simulink model "AFC_FFNN_trainlm_15_15_15_15_Apr_1_2020"  (R2022b)
settings: Solver=ode15s  StartTime=0.0  StopTime=T  MaxStep=.01  RelTol=1e-3
undefined symbols (not defined in the file): AF_sensor_tol, fault_time, fuel_inj_tol, kappa_tol, MAF_sensor_tol, pump_tol, tau_ww_tol
libraries: neural x66
(part 2 of 3)

== system AFC_FFNN_trainlm_15_15_15_15_Apr_1_2020/Air Fuel Control Model 1/Feed-Forward Neural Network/Layer 2/Delays 1 ==
  "p{2}" : Inport  PortDimensions=15
      mask Display: e = 0.06;c1 = [120 230 180]/255;c2 = ([120 230 180]+0)/(256+128);c3 = ([120 230 180]+128)/(256+128);patch([0 1 1 0],[0 0 1 1],c1);patch([0 1 1 1-e 1-e 0+e],[0 0 1 1-e 0+e 0+e],c2);patch([0 0 1 1-e 0+e 0+e],[0 1 1 1-e 1-e 0+e],c3);plot([0 1 1 0 0],[0 0 1 1 0]);
  mux : Mux  Inputs=1
      mask Display: e = 0.06;c1 = [120 150 230]/255;c2 = ([120 150 230]+0)/383;c3 = ([120 150 230]+128)/383;patch([0 1 1 0],[0 0 1 1],c1);patch([0 1 1 1-e 1-e 0+e],[0 0 1 1-e 0+e 0+e],c2);patch([0 0 1 1-e 0+e 0+e],[0 1 1 1-e 1-e 0+e],c3);plot([0 1 1 0 0],[0 0 1 1 0]);disp('Mux')
  "pd{2,1}" : Outport
      mask Display: e = 0.06;c1 = [120 230 180]/255;c2 = ([120 230 180]+0)/(256+128);c3 = ([120 230 180]+128)/(256+128);patch([0 1 1 0],[0 0 1 1],c1);patch([0 1 1 1-e 1-e 0+e],[0 0 1 1-e 0+e 0+e],c2);patch([0 0 1 1-e 0+e 0+e],[0 1 1 1-e 1-e 0+e],c3);plot([0 1 1 0 0],[0 0 1 1 0]);
  wires:
  "p{2}"/1 -> mux/1
  mux/1 -> "pd{2,1}"/1

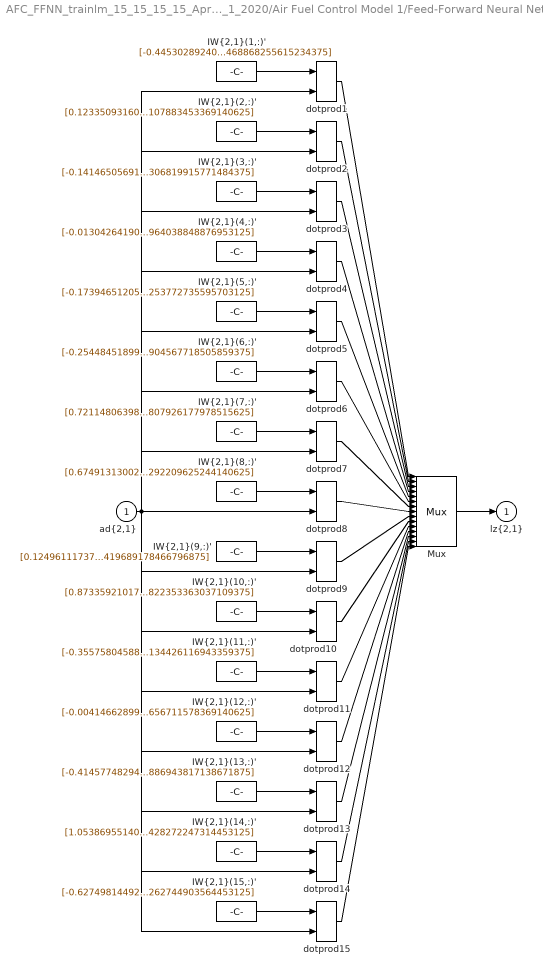
== system AFC_FFNN_trainlm_15_15_15_15_Apr_1_2020/Air Fuel Control Model 1/Feed-Forward Neural Network/Layer 2/LW{2,1} ==
  "ad{2,1}" : Inport  PortDimensions=15
      mask Display: e = 0.06;c1 = [120 230 180]/255;c2 = ([120 230 180]+0)/(256+128);c3 = ([120 230 180]+128)/(256+128);patch([0 1 1 0],[0 0 1 1],c1);patch([0 1 1 1-e 1-e 0+e],[0 0 1 1-e 0+e 0+e],c2);patch([0 0 1 1-e 0+e 0+e],[0 1 1 1-e 1-e 0+e],c3);plot([0 1 1 0 0],[0 0 1 1 0]);
  "IW{2,1}(1,:)'" : Constant  Value=[-0.44530289240325071631332320976071059703826904296875;-0.031599090975333421482673657010309398174285888671875;-0.9859158830932484018916284185252152383327484130859375;0.83077856260949634048529333085753023624420166015625;0.5147405056908984644081783699220977723598480224609375;-0.59941875528171539855293303844518959522247314453125;-0.9340218456622333409455904984497465193271636962890625;-0.2001276258897833615346684155156253837049007415771484375;0.08055251588838825693716927389687043614685535430908203125;-0.6770620370683728683758317856700159609317779541015625;0.318318052739778700743755734947626478970050811767578125;-0.51093086630106798740058593466528691351413726806640625;-0.44231337771352940979596723991562612354755401611328125;0.445164828909296483860913440366857685148715972900390625;0.9246634629628525114952708463533781468868255615234375]
      mask Display: e = 0.06;c1 = [120 150 230]/255;c2 = ([120 150 230]+0)/383;c3 = ([120 150 230]+128)/383;patch([0 1 1 0],[0 0 1 1],c1);patch([0 1 1 1-e 1-e 0+e],[0 0 1 1-e 0+e 0+e],c2);patch([0 0 1 1-e 0+e 0+e],[0 1 1 1-e 1-e 0+e],c3);plot([0 1 1 0 0],[0 0 1 1 0]);disp('weights');
  "IW{2,1}(10,:)'" : Constant  Value=[0.87335921017074824579395908585865981876850128173828125;0.3045430612282420401726312775281257927417755126953125;0.2262366289036867872397351675317622721195220947265625;-0.0737735854276786173766566889753448776900768280029296875;-0.63864720704534294615228873226442374289035797119140625;0.2937771056857114704286004780442453920841217041015625;0.56879031291023995908773258634028024971485137939453125;0.8502258695783304620618991975788958370685577392578125;0.59046290655221811416453192578046582639217376708984375;0.742343450952053895974813713110052049160003662109375;0.330116034595487717329120869180769659578800201416015625;0.422958081116346085170931701213703490793704986572265625;-0.5932782732724366514531766370055265724658966064453125;0.24289284049794712672110108542256057262420654296875;0.0864280836636444060872008776641450822353363037109375]
      mask Display: e = 0.06;c1 = [120 150 230]/255;c2 = ([120 150 230]+0)/383;c3 = ([120 150 230]+128)/383;patch([0 1 1 0],[0 0 1 1],c1);patch([0 1 1 1-e 1-e 0+e],[0 0 1 1-e 0+e 0+e],c2);patch([0 0 1 1-e 0+e 0+e],[0 1 1 1-e 1-e 0+e],c3);plot([0 1 1 0 0],[0 0 1 1 0]);disp('weights');
  "IW{2,1}(11,:)'" : Constant  Value=[-0.355758045882987428143451325013302266597747802734375;0.95738371421368118063810470630414783954620361328125;-0.045379138797660534265787646290846168994903564453125;-0.09801334374643477787003575940616428852081298828125;-0.918603047640635939075082205818034708499908447265625;-0.8674218274916183357703403089544735848903656005859375;-0.6442562627279382336809021580847911536693572998046875;-0.5798997854751615221857719006948173046112060546875;-0.268117521648080892049392787157557904720306396484375;-0.386098950836792909058203804306685924530029296875;-0.250737493036341962948654327192343771457672119140625;0.19542355542480294161578058265149593353271484375;-0.3831562328000919226411724594072438776493072509765625;-0.5144921285647086062198241052101366221904754638671875;0.4519361428046548834203122169128619134426116943359375]
      mask Display: e = 0.06;c1 = [120 150 230]/255;c2 = ([120 150 230]+0)/383;c3 = ([120 150 230]+128)/383;patch([0 1 1 0],[0 0 1 1],c1);patch([0 1 1 1-e 1-e 0+e],[0 0 1 1-e 0+e 0+e],c2);patch([0 0 1 1-e 0+e 0+e],[0 1 1 1-e 1-e 0+e],c3);plot([0 1 1 0 0],[0 0 1 1 0]);disp('weights');
  "IW{2,1}(12,:)'" : Constant  Value=[-0.00414662899800699591423835954628884792327880859375;-0.9036999234519438317647654912434518337249755859375;-0.608291622828492251073839724995195865631103515625;-0.2562202759423455322718155002803541719913482666015625;-0.4269761403475114125427580802352167665958404541015625;0.194105158589592985407534797559492290019989013671875;0.536814598299950151982784518622793257236480712890625;0.51556253517868289026893080517766065895557403564453125;-0.9952187767754754332827360485680401325225830078125;-0.2577903717954541651380395705928094685077667236328125;-0.6898788629360759205866315824096091091632843017578125;-0.2222878005231464226820747853707871399819850921630859375;0.297875717286642416326003512949682772159576416015625;-0.7508353369592175585722770847496576607227325439453125;-0.50523180372987841479925918974913656711578369140625]
      mask Display: e = 0.06;c1 = [120 150 230]/255;c2 = ([120 150 230]+0)/383;c3 = ([120 150 230]+128)/383;patch([0 1 1 0],[0 0 1 1],c1);patch([0 1 1 1-e 1-e 0+e],[0 0 1 1-e 0+e 0+e],c2);patch([0 0 1 1-e 0+e 0+e],[0 1 1 1-e 1-e 0+e],c3);plot([0 1 1 0 0],[0 0 1 1 0]);disp('weights');
  "IW{2,1}(13,:)'" : Constant  Value=[-0.4145774829441866149437601052341051399707794189453125;0.14729631413513910587198552093468606472015380859375;0.270210509357474482072802857146598398685455322265625;0.57010688508284845799067852567532099783420562744140625;-0.8414780044291469973671837578876875340938568115234375;0.9203189787835868163057284618844278156757354736328125;-0.4843710655220123673103671535500325262546539306640625;-1.0675012319238594837855771402246318757534027099609375;-0.320838849990772556619589295223704539239406585693359375;0.9873821817269874401290508103556931018829345703125;0.54849877750004727428034811964607797563076019287109375;0.569544378285404828687887857086025178432464599609375;0.2108285610691495171042930678595439530909061431884765625;0.06983728871402901383635963838969473727047443389892578125;0.8840117899428008296780490127275697886943817138671875]
      mask Display: e = 0.06;c1 = [120 150 230]/255;c2 = ([120 150 230]+0)/383;c3 = ([120 150 230]+128)/383;patch([0 1 1 0],[0 0 1 1],c1);patch([0 1 1 1-e 1-e 0+e],[0 0 1 1-e 0+e 0+e],c2);patch([0 0 1 1-e 0+e 0+e],[0 1 1 1-e 1-e 0+e],c3);plot([0 1 1 0 0],[0 0 1 1 0]);disp('weights');
  "IW{2,1}(14,:)'" : Constant  Value=[1.053869551407217830529816637863405048847198486328125;0.3528287446453199915907816830440424382686614990234375;-0.09371681637081774596254035714082419872283935546875;-0.76902743658348515776168596858042292296886444091796875;0.58884882984626363278124472344643436372280120849609375;0.782969545193491711643218877725303173065185546875;0.8048470896960198128766705849557183682918548583984375;-0.1666021907992077666360586363225593231618404388427734375;-0.1625558961280517689118596535990945994853973388671875;-0.0742329299648212259654656008933670818805694580078125;0.96503755663264667585821143802604638040065765380859375;0.1873196926068718681790414848364889621734619140625;0.197095112469012734290885191512643359601497650146484375;0.0776951180269920549381623686713282950222492218017578125;-0.1032133985101542084095171958324499428272247314453125]
      mask Display: e = 0.06;c1 = [120 150 230]/255;c2 = ([120 150 230]+0)/383;c3 = ([120 150 230]+128)/383;patch([0 1 1 0],[0 0 1 1],c1);patch([0 1 1 1-e 1-e 0+e],[0 0 1 1-e 0+e 0+e],c2);patch([0 0 1 1-e 0+e 0+e],[0 1 1 1-e 1-e 0+e],c3);plot([0 1 1 0 0],[0 0 1 1 0]);disp('weights');
  "IW{2,1}(15,:)'" : Constant  Value=[-0.62749814492342348426490161727997474372386932373046875;-0.6065698611977108356541066314093768596649169921875;-0.5498532544670771127215402884758077561855316162109375;-0.446263434355464172487160112723358906805515289306640625;-0.53706583703445431865475256927311420440673828125;-0.0280657246307758345693628143635578453540802001953125;0.417070734839645684832731831193086691200733184814453125;-0.5109740241601594679110576180391944944858551025390625;0.73027841342623756037966131771099753677845001220703125;0.8030937049055861809421230645966716110706329345703125;0.140951156143085232219647195961442776024341583251953125;-0.6225469098087774710847952519543468952178955078125;0.7234673765292074509858366582193411886692047119140625;-0.08109737982096669461906657261351938359439373016357421875;-0.3366599736262987363488718983717262744903564453125]
      mask Display: e = 0.06;c1 = [120 150 230]/255;c2 = ([120 150 230]+0)/383;c3 = ([120 150 230]+128)/383;patch([0 1 1 0],[0 0 1 1],c1);patch([0 1 1 1-e 1-e 0+e],[0 0 1 1-e 0+e 0+e],c2);patch([0 0 1 1-e 0+e 0+e],[0 1 1 1-e 1-e 0+e],c3);plot([0 1 1 0 0],[0 0 1 1 0]);disp('weights');
  "IW{2,1}(2,:)'" : Constant  Value=[0.123350931609165659352811417193152010440826416015625;0.864528436490474394560123982955701649188995361328125;0.335475936157511700486111294594593346118927001953125;-0.5899507915690425097210436433670111000537872314453125;-0.73320113507208695136085907506640069186687469482421875;0.23542378407344433099979141843505203723907470703125;-1.2983368068898675229405625941581092774868011474609375;-0.46114795420050480601048548123799264430999755859375;-0.6295420404604257225145147458533756434917449951171875;-0.111941927115701833628236272488720715045928955078125;0.17752782398035105160261082346551120281219482421875;0.0004416803790633083703909278483479283750057220458984375;-0.8155097377306848027700425518560223281383514404296875;-0.393416725481041285039651711485930718481540679931640625;-0.1554515399646947404477259624400176107883453369140625]
      mask Display: e = 0.06;c1 = [120 150 230]/255;c2 = ([120 150 230]+0)/383;c3 = ([120 150 230]+128)/383;patch([0 1 1 0],[0 0 1 1],c1);patch([0 1 1 1-e 1-e 0+e],[0 0 1 1-e 0+e 0+e],c2);patch([0 0 1 1-e 0+e 0+e],[0 1 1 1-e 1-e 0+e],c3);plot([0 1 1 0 0],[0 0 1 1 0]);disp('weights');
  "IW{2,1}(3,:)'" : Constant  Value=[-0.141465056911737774303361447891802527010440826416015625;-0.5154584472501750891382243935368023812770843505859375;0.9439746204251926453565602059825323522090911865234375;0.75078355276593489175951390279806219041347503662109375;-0.447927632287961230428408043735544197261333465576171875;0.474517977902461751682494650594890117645263671875;-0.01018244174709355409635946898561087436974048614501953125;-0.8638553713183194648905782742076553404331207275390625;-0.00964066360971845004446123539310065098106861114501953125;0.326326978715826054866511185537092387676239013671875;-0.75409103785881914649991131227579899132251739501953125;0.5359710901816538974884451818070374429225921630859375;0.1424466067912671107809075010663946159183979034423828125;0.2092469885290515752007678429436055012047290802001953125;-0.275716837344263776543584754108451306819915771484375]
      mask Display: e = 0.06;c1 = [120 150 230]/255;c2 = ([120 150 230]+0)/383;c3 = ([120 150 230]+128)/383;patch([0 1 1 0],[0 0 1 1],c1);patch([0 1 1 1-e 1-e 0+e],[0 0 1 1-e 0+e 0+e],c2);patch([0 0 1 1-e 0+e 0+e],[0 1 1 1-e 1-e 0+e],c3);plot([0 1 1 0 0],[0 0 1 1 0]);disp('weights');
  "IW{2,1}(4,:)'" : Constant  Value=[-0.01304264190607866413795790094809490256011486053466796875;0.5008207528485264514728214635397307574748992919921875;0.5232965506775359987301499131717719137668609619140625;-0.4811450968966723973352372922818176448345184326171875;-1.0049682257868945978174224364920519292354583740234375;0.4799582216277162860507132791099138557910919189453125;0.73297744388027552542297371473978273570537567138671875;-0.84040208853851072756668827423709444701671600341796875;0.181024008721385298859019030714989639818668365478515625;0.946413330197788837949701701290905475616455078125;0.10731012634836163688323296128146466799080371856689453125;-0.307975119967440258417212817221297882497310638427734375;0.261780874000085594932585308924899436533451080322265625;0.59747952306587504001100796813261695206165313720703125;-0.554550225837776356030417446163482964038848876953125]
      mask Display: e = 0.06;c1 = [120 150 230]/255;c2 = ([120 150 230]+0)/383;c3 = ([120 150 230]+128)/383;patch([0 1 1 0],[0 0 1 1],c1);patch([0 1 1 1-e 1-e 0+e],[0 0 1 1-e 0+e 0+e],c2);patch([0 0 1 1-e 0+e 0+e],[0 1 1 1-e 1-e 0+e],c3);plot([0 1 1 0 0],[0 0 1 1 0]);disp('weights');
  "IW{2,1}(5,:)'" : Constant  Value=[-0.1739465120590377722464836551807820796966552734375;-0.4253934049515246673678348088287748396396636962890625;0.107688842394002559643695349222980439662933349609375;-0.81164996832045444019598789964220486581325531005859375;0.55762116856230126149540637925383634865283966064453125;-0.636255188237751401203468049061484634876251220703125;-0.74211277790886054361862989026121795177459716796875;0.00119064586918475601162725752146798186004161834716796875;-0.928692502411525566685668309219181537628173828125;0.8916047859232898442627401891513727605342864990234375;0.5140824228731524225821658546919934451580047607421875;0.4896657104983976882550678055849857628345489501953125;-0.720566800434029541833069743006490170955657958984375;-0.3805195389795958949008536364999599754810333251953125;0.3718653345102265195265545116853900253772735595703125]
      mask Display: e = 0.06;c1 = [120 150 230]/255;c2 = ([120 150 230]+0)/383;c3 = ([120 150 230]+128)/383;patch([0 1 1 0],[0 0 1 1],c1);patch([0 1 1 1-e 1-e 0+e],[0 0 1 1-e 0+e 0+e],c2);patch([0 0 1 1-e 0+e 0+e],[0 1 1 1-e 1-e 0+e],c3);plot([0 1 1 0 0],[0 0 1 1 0]);disp('weights');
  "IW{2,1}(6,:)'" : Constant  Value=[-0.2544845189978541810660317423753440380096435546875;0.331236793833797005248698042123578488826751708984375;-0.2650153662478154092951854181592352688312530517578125;-0.8030108697323161681680403489735908806324005126953125;-0.0809935269792434464619645950733684003353118896484375;-0.3458413777341948769361579252290539443492889404296875;0.5797107755346486701597541468800045549869537353515625;-0.3924755511796911289223999119712971150875091552734375;0.0862249490760589321070028745452873408794403076171875;0.3349078583902673766914404041017405688762664794921875;-0.670848103624811731293675620690919458866119384765625;0.7692397856389321386672008884488604962825775146484375;-0.1385671931480672025571720951120369136333465576171875;-0.86550241542650940829162209411151707172393798828125;0.0620399548241079568100531105301342904567718505859375]
      mask Display: e = 0.06;c1 = [120 150 230]/255;c2 = ([120 150 230]+0)/383;c3 = ([120 150 230]+128)/383;patch([0 1 1 0],[0 0 1 1],c1);patch([0 1 1 1-e 1-e 0+e],[0 0 1 1-e 0+e 0+e],c2);patch([0 0 1 1-e 0+e 0+e],[0 1 1 1-e 1-e 0+e],c3);plot([0 1 1 0 0],[0 0 1 1 0]);disp('weights');
  "IW{2,1}(7,:)'" : Constant  Value=[0.72114806398727815395233164963428862392902374267578125;-0.978377493020309518811927773640491068363189697265625;0.0643583126957845141902225805097259581089019775390625;-0.67897862057058144813481703749857842922210693359375;0.66980541326278586478082388566690497100353240966796875;-0.0354769119507334362850770048680715262889862060546875;-0.357660668445020479833118542956071905791759490966796875;-0.9527975809755375724563464245875366032123565673828125;0.492191119953068689785169453898561187088489532470703125;-0.3817584213426652439693498308770358562469482421875;0.83261624191043337450679473477066494524478912353515625;-0.1348669419743790676147199292245204560458660125732421875;-0.09933470153220687326456328491985914297401905059814453125;0.67479085648442593825535595897235907614231109619140625;-0.17542651465642311592318947077728807926177978515625]
      mask Display: e = 0.06;c1 = [120 150 230]/255;c2 = ([120 150 230]+0)/383;c3 = ([120 150 230]+128)/383;patch([0 1 1 0],[0 0 1 1],c1);patch([0 1 1 1-e 1-e 0+e],[0 0 1 1-e 0+e 0+e],c2);patch([0 0 1 1-e 0+e 0+e],[0 1 1 1-e 1-e 0+e],c3);plot([0 1 1 0 0],[0 0 1 1 0]);disp('weights');
  "IW{2,1}(8,:)'" : Constant  Value=[0.674913130028367280743850642465986311435699462890625;-0.7740439681869883958853506555897183716297149658203125;0.3677008538220587485767509861034341156482696533203125;-0.2438667636767749280490846786051406525075435638427734375;-0.12026647773071998115401726181517005898058414459228515625;0.6386910988199769878548295309883542358875274658203125;0.71707718927074048931302741038962267339229583740234375;0.4826744554070157011693709137034602463245391845703125;-0.724201667967991458141341354348696768283843994140625;-0.4870732286702981195247730283881537616252899169921875;0.6329643952082069091602534172125160694122314453125;0.1929886494914454519999935655505396425724029541015625;-0.55148303333209780507928599035949446260929107666015625;-0.445425365212919588397966208503930829465389251708984375;0.9911239400503648599993766765692271292209625244140625]
      mask Display: e = 0.06;c1 = [120 150 230]/255;c2 = ([120 150 230]+0)/383;c3 = ([120 150 230]+128)/383;patch([0 1 1 0],[0 0 1 1],c1);patch([0 1 1 1-e 1-e 0+e],[0 0 1 1-e 0+e 0+e],c2);patch([0 0 1 1-e 0+e 0+e],[0 1 1 1-e 1-e 0+e],c3);plot([0 1 1 0 0],[0 0 1 1 0]);disp('weights');
  "IW{2,1}(9,:)'" : Constant  Value=[0.1249611173784332673886154907449963502585887908935546875;0.9997366417680042527393879936425946652889251708984375;-0.4060487137094297427353239982039667665958404541015625;-0.6678251770476755222460951699758879840373992919921875;0.476779894257461422935051587046473287045955657958984375;0.748692070069837622980912783532403409481048583984375;0.71619942289555338366113801384926773607730865478515625;0.681501358673081814032457259600050747394561767578125;-0.313516269761654087222524367462028749287128448486328125;0.9408656718724746070847686496563255786895751953125;-0.51092205682236124797412912812433205544948577880859375;0.474973316386256116938824334283708594739437103271484375;0.4967103873360889654264838100061751902103424072265625;0.1966063607784174493975370978660066612064838409423828125;-0.602322264728701650682296531158499419689178466796875]
      mask Display: e = 0.06;c1 = [120 150 230]/255;c2 = ([120 150 230]+0)/383;c3 = ([120 150 230]+128)/383;patch([0 1 1 0],[0 0 1 1],c1);patch([0 1 1 1-e 1-e 0+e],[0 0 1 1-e 0+e 0+e],c2);patch([0 0 1 1-e 0+e 0+e],[0 1 1 1-e 1-e 0+e],c3);plot([0 1 1 0 0],[0 0 1 1 0]);disp('weights');
  Mux : Mux  Inputs=15
      mask Display: e = 0.06;c1 = [120 150 230]/255;c2 = ([120 150 230]+0)/383;c3 = ([120 150 230]+128)/383;patch([0 1 1 0],[0 0 1 1],c1);patch([0 1 1 1-e 1-e 0+e],[0 0 1 1-e 0+e 0+e],c2);patch([0 0 1 1-e 0+e 0+e],[0 1 1 1-e 1-e 0+e],c3);plot([0 1 1 0 0],[0 0 1 1 0]);disp('Mux');
  dotprod{1..15} (15 alike) : neural/Weight Functions/dotprod
  "lz{2,1}" : Outport
      mask Display: e = 0.06;c1 = [120 230 180]/255;c2 = ([120 230 180]+0)/(256+128);c3 = ([120 230 180]+128)/(256+128);patch([0 1 1 0],[0 0 1 1],c1);patch([0 1 1 1-e 1-e 0+e],[0 0 1 1-e 0+e 0+e],c2);patch([0 0 1 1-e 0+e 0+e],[0 1 1 1-e 1-e 0+e],c3);plot([0 1 1 0 0],[0 0 1 1 0]);
  wires:
  "IW{2,1}(1,:)'"/1 -> dotprod1/1
  "ad{2,1}"/1 -> dotprod1/2, dotprod2/2, dotprod3/2, dotprod4/2, dotprod5/2, dotprod6/2, dotprod7/2, dotprod8/2, dotprod9/2, dotprod10/2, dotprod11/2, dotprod12/2, dotprod13/2, dotprod14/2, dotprod15/2
  dotprod1/1 -> Mux/1
  "IW{2,1}(2,:)'"/1 -> dotprod2/1
  dotprod2/1 -> Mux/2
  "IW{2,1}(3,:)'"/1 -> dotprod3/1
  dotprod3/1 -> Mux/3
  "IW{2,1}(4,:)'"/1 -> dotprod4/1
  dotprod4/1 -> Mux/4
  "IW{2,1}(5,:)'"/1 -> dotprod5/1
  dotprod5/1 -> Mux/5
  "IW{2,1}(6,:)'"/1 -> dotprod6/1
  dotprod6/1 -> Mux/6
  "IW{2,1}(7,:)'"/1 -> dotprod7/1
  dotprod7/1 -> Mux/7
  "IW{2,1}(8,:)'"/1 -> dotprod8/1
  dotprod8/1 -> Mux/8
  "IW{2,1}(9,:)'"/1 -> dotprod9/1
  dotprod9/1 -> Mux/9
  "IW{2,1}(10,:)'"/1 -> dotprod10/1
  dotprod10/1 -> Mux/10
  "IW{2,1}(11,:)'"/1 -> dotprod11/1
  dotprod11/1 -> Mux/11
  "IW{2,1}(12,:)'"/1 -> dotprod12/1
  dotprod12/1 -> Mux/12
  "IW{2,1}(13,:)'"/1 -> dotprod13/1
  dotprod13/1 -> Mux/13
  "IW{2,1}(14,:)'"/1 -> dotprod14/1
  dotprod14/1 -> Mux/14
  "IW{2,1}(15,:)'"/1 -> dotprod15/1
  dotprod15/1 -> Mux/15
  Mux/1 -> "lz{2,1}"/1

== system AFC_FFNN_trainlm_15_15_15_15_Apr_1_2020/Air Fuel Control Model 1/Feed-Forward Neural Network/Layer 3/Delays 1 ==
  "p{3}" : Inport  PortDimensions=15
      mask Display: e = 0.06;c1 = [120 230 180]/255;c2 = ([120 230 180]+0)/(256+128);c3 = ([120 230 180]+128)/(256+128);patch([0 1 1 0],[0 0 1 1],c1);patch([0 1 1 1-e 1-e 0+e],[0 0 1 1-e 0+e 0+e],c2);patch([0 0 1 1-e 0+e 0+e],[0 1 1 1-e 1-e 0+e],c3);plot([0 1 1 0 0],[0 0 1 1 0]);
  mux : Mux  Inputs=1
      mask Display: e = 0.06;c1 = [120 150 230]/255;c2 = ([120 150 230]+0)/383;c3 = ([120 150 230]+128)/383;patch([0 1 1 0],[0 0 1 1],c1);patch([0 1 1 1-e 1-e 0+e],[0 0 1 1-e 0+e 0+e],c2);patch([0 0 1 1-e 0+e 0+e],[0 1 1 1-e 1-e 0+e],c3);plot([0 1 1 0 0],[0 0 1 1 0]);disp('Mux')
  "pd{3,2}" : Outport
      mask Display: e = 0.06;c1 = [120 230 180]/255;c2 = ([120 230 180]+0)/(256+128);c3 = ([120 230 180]+128)/(256+128);patch([0 1 1 0],[0 0 1 1],c1);patch([0 1 1 1-e 1-e 0+e],[0 0 1 1-e 0+e 0+e],c2);patch([0 0 1 1-e 0+e 0+e],[0 1 1 1-e 1-e 0+e],c3);plot([0 1 1 0 0],[0 0 1 1 0]);
  wires:
  "p{3}"/1 -> mux/1
  mux/1 -> "pd{3,2}"/1

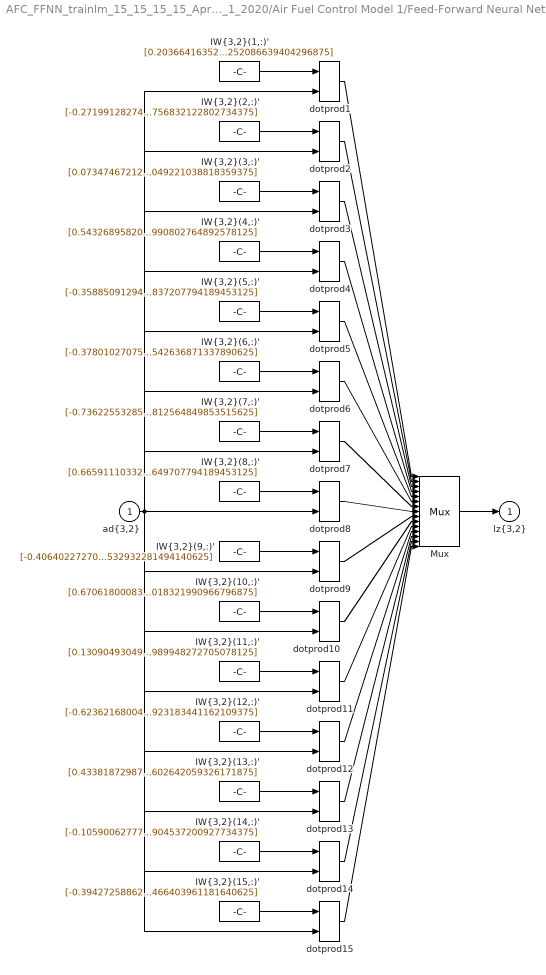
== system AFC_FFNN_trainlm_15_15_15_15_Apr_1_2020/Air Fuel Control Model 1/Feed-Forward Neural Network/Layer 3/LW{3,2} ==
  "ad{3,2}" : Inport  PortDimensions=15
      mask Display: e = 0.06;c1 = [120 230 180]/255;c2 = ([120 230 180]+0)/(256+128);c3 = ([120 230 180]+128)/(256+128);patch([0 1 1 0],[0 0 1 1],c1);patch([0 1 1 1-e 1-e 0+e],[0 0 1 1-e 0+e 0+e],c2);patch([0 0 1 1-e 0+e 0+e],[0 1 1 1-e 1-e 0+e],c3);plot([0 1 1 0 0],[0 0 1 1 0]);
  "IW{3,2}(1,:)'" : Constant  Value=[0.203664163529512387551534402518882416188716888427734375;-0.3003049887536757278638788193347863852977752685546875;0.6906714609452382358512068094569258391857147216796875;-0.83087046120422336503708038435433991253376007080078125;-0.71632698966811203522553341827006079256534576416015625;-0.3582382310064227137758052776916883885860443115234375;0.8217795233401357091196359760942868888378143310546875;-0.34470671555417398135290341087966226041316986083984375;0.2199805944249561273640125591555261053144931793212890625;-0.8022103686807129374614078187732957303524017333984375;0.455030961948063694677557577961124479770660400390625;-0.5999825945944790017705372520140372216701507568359375;0.1153881623794226485291147810130496509373188018798828125;0.69062856984264897608483124713529832661151885986328125;-0.263508173547184643137342163754510693252086639404296875]
      mask Display: e = 0.06;c1 = [120 150 230]/255;c2 = ([120 150 230]+0)/383;c3 = ([120 150 230]+128)/383;patch([0 1 1 0],[0 0 1 1],c1);patch([0 1 1 1-e 1-e 0+e],[0 0 1 1-e 0+e 0+e],c2);patch([0 0 1 1-e 0+e 0+e],[0 1 1 1-e 1-e 0+e],c3);plot([0 1 1 0 0],[0 0 1 1 0]);disp('weights');
  "IW{3,2}(10,:)'" : Constant  Value=[0.67061800083705025432578850086429156363010406494140625;-0.03920815403831279244428742458694614470005035400390625;-0.36943253195595193716371795744635164737701416015625;-0.134042988062515633362892231161822564899921417236328125;-0.73636359128011530383872695892932824790477752685546875;-0.0955593194571180415408662156551145017147064208984375;0.7674384556721578487525903256027959287166595458984375;0.6149679765232602957070184857002459466457366943359375;0.01230575834134401726205343408082626410759985446929931640625;-0.67408758124629331032195977968513034284114837646484375;0.4752439715777379003469604867859743535518646240234375;-1.09001582772559491019137567491270601749420166015625;-0.265979995412270853183400731722940690815448760986328125;0.925497608964296336608867932227440178394317626953125;-0.1449623016588758861455943360851961188018321990966796875]
      mask Display: e = 0.06;c1 = [120 150 230]/255;c2 = ([120 150 230]+0)/383;c3 = ([120 150 230]+128)/383;patch([0 1 1 0],[0 0 1 1],c1);patch([0 1 1 1-e 1-e 0+e],[0 0 1 1-e 0+e 0+e],c2);patch([0 0 1 1-e 0+e 0+e],[0 1 1 1-e 1-e 0+e],c3);plot([0 1 1 0 0],[0 0 1 1 0]);disp('weights');
  "IW{3,2}(11,:)'" : Constant  Value=[0.13090493049776530387617867745575495064258575439453125;0.8789214887799270403689888553344644606113433837890625;0.498002993921559722334535535992472432553768157958984375;-0.520697815088529747384882284677587449550628662109375;0.969461790374972043338175353710539638996124267578125;-0.3153616709473954227149761209147982299327850341796875;0.07963378051882634423019879932326148264110088348388671875;0.60494069742346512352781928711920045316219329833984375;-0.55848491080131967834176975884474813938140869140625;-1.6101561463982794197846715178457088768482208251953125;0.482059004928104162246427222271449863910675048828125;-0.067041856006378408583401551368297077715396881103515625;0.68798704870989280113491304291528649628162384033203125;-1.025985627803987387807183040422387421131134033203125;0.64060415796041347835654278242145664989948272705078125]
      mask Display: e = 0.06;c1 = [120 150 230]/255;c2 = ([120 150 230]+0)/383;c3 = ([120 150 230]+128)/383;patch([0 1 1 0],[0 0 1 1],c1);patch([0 1 1 1-e 1-e 0+e],[0 0 1 1-e 0+e 0+e],c2);patch([0 0 1 1-e 0+e 0+e],[0 1 1 1-e 1-e 0+e],c3);plot([0 1 1 0 0],[0 0 1 1 0]);disp('weights');
  "IW{3,2}(12,:)'" : Constant  Value=[-0.623621680045882254006528455647639930248260498046875;0.745786236117528478217764131841249763965606689453125;0.395873623849920808215330225721118040382862091064453125;-0.394229471877415083014284391538240015506744384765625;0.02174067578361071895187706104479730129241943359375;-0.8911737617128647759301429687184281647205352783203125;-0.0764583990603655561102414139895699918270111083984375;0.6467406928718426595281698610051535069942474365234375;0.06909886567012468727710938765085302293300628662109375;0.27153060848236887370177328193676657974720001220703125;0.63467246646910968621568827074952423572540283203125;-0.444826066560185251486103652496240101754665374755859375;-0.045679511305048270397577425683266483247280120849609375;-0.301505432149076657566411086008884012699127197265625;-0.823404274767673083346153362072072923183441162109375]
      mask Display: e = 0.06;c1 = [120 150 230]/255;c2 = ([120 150 230]+0)/383;c3 = ([120 150 230]+128)/383;patch([0 1 1 0],[0 0 1 1],c1);patch([0 1 1 1-e 1-e 0+e],[0 0 1 1-e 0+e 0+e],c2);patch([0 0 1 1-e 0+e 0+e],[0 1 1 1-e 1-e 0+e],c3);plot([0 1 1 0 0],[0 0 1 1 0]);disp('weights');
  "IW{3,2}(13,:)'" : Constant  Value=[0.4338187298798230617791205077082850039005279541015625;0.036406136205346939505034242756664752960205078125;-0.0473174293087244013378267482039518654346466064453125;0.0896110097964906149314856520504690706729888916015625;-0.468632007291200469722980415099300444126129150390625;-0.1261809277287484487573010483174584805965423583984375;-0.842109691431418116991380884428508579730987548828125;0.6107811321229810186395070559228770434856414794921875;-0.4289594236134040006191980864969082176685333251953125;-0.1345071670124424745296209948719479143619537353515625;-0.2360527622534238645357618224807083606719970703125;0.865730871275315561064189751050435006618499755859375;-0.9688229942094033209087911018286831676959991455078125;-0.881570871778942777297061184071935713291168212890625;0.912409898058981649882070996682159602642059326171875]
      mask Display: e = 0.06;c1 = [120 150 230]/255;c2 = ([120 150 230]+0)/383;c3 = ([120 150 230]+128)/383;patch([0 1 1 0],[0 0 1 1],c1);patch([0 1 1 1-e 1-e 0+e],[0 0 1 1-e 0+e 0+e],c2);patch([0 0 1 1-e 0+e 0+e],[0 1 1 1-e 1-e 0+e],c3);plot([0 1 1 0 0],[0 0 1 1 0]);disp('weights');
  "IW{3,2}(14,:)'" : Constant  Value=[-0.105900627771794819675932330937939696013927459716796875;-0.78609897524188721007476488011889159679412841796875;-0.382919018789930287738343395176343619823455810546875;-0.49611957369466974654415025725029408931732177734375;0.6589169152345280000560023836442269384860992431640625;0.27840929729416696858379509649239480495452880859375;-0.7675632445112829937983178751892410218715667724609375;0.40879670598666117964370414483710192143917083740234375;0.0221429075001386699295125026765163056552410125732421875;0.05342048065787392829850688258375157602131366729736328125;-0.0413625689516228245423690168536268174648284912109375;-0.0659170156870927670400561737551470287144184112548828125;-0.467794761040074724700588149062241427600383758544921875;-0.501956085840327137503891208325512707233428955078125;0.7310507035321955893181211649789474904537200927734375]
      mask Display: e = 0.06;c1 = [120 150 230]/255;c2 = ([120 150 230]+0)/383;c3 = ([120 150 230]+128)/383;patch([0 1 1 0],[0 0 1 1],c1);patch([0 1 1 1-e 1-e 0+e],[0 0 1 1-e 0+e 0+e],c2);patch([0 0 1 1-e 0+e 0+e],[0 1 1 1-e 1-e 0+e],c3);plot([0 1 1 0 0],[0 0 1 1 0]);disp('weights');
  "IW{3,2}(15,:)'" : Constant  Value=[-0.394272588629856646225135818895068950951099395751953125;0.365980954055685148151866314947255887091159820556640625;-0.715600617274316785909604732296429574489593505859375;0.26173793147083745935788101633079349994659423828125;0.289378575464602605382680167167563922703266143798828125;-0.155364445914564885953268458251841366291046142578125;-0.6543215518736211766537280709599144756793975830078125;-40740.48239736151299439370632171630859375;-0.38426447232318705626852306522778235375881195068359375;0.697843570401849522255588453845120966434478759765625;-0.766330988753066488783360910019837319850921630859375;-4.02765264084377516695667509338818490505218505859375;-0.518307771496965496993425404070876538753509521484375;-0.8002212397643939656433076379471458494663238525390625;-0.82050982696684915396190262981690466403961181640625]
      mask Display: e = 0.06;c1 = [120 150 230]/255;c2 = ([120 150 230]+0)/383;c3 = ([120 150 230]+128)/383;patch([0 1 1 0],[0 0 1 1],c1);patch([0 1 1 1-e 1-e 0+e],[0 0 1 1-e 0+e 0+e],c2);patch([0 0 1 1-e 0+e 0+e],[0 1 1 1-e 1-e 0+e],c3);plot([0 1 1 0 0],[0 0 1 1 0]);disp('weights');
  "IW{3,2}(2,:)'" : Constant  Value=[-0.27199128274895112422626652914914302527904510498046875;0.59112467210576280507439150824211537837982177734375;0.02211883911810240410655836740261293016374111175537109375;-0.7125931940952952015067012325744144618511199951171875;0.67616899571989208528322023994405753910541534423828125;-0.6999107897552205859170726398588158190250396728515625;-0.62995073687626479408407931259716860949993133544921875;0.76272989777451372095384840577025897800922393798828125;0.025018201027044495443618643548688851296901702880859375;0.7437540465053145144480595263303257524967193603515625;0.3710457681335530555344348613289184868335723876953125;0.62745425052057768322555375561933033168315887451171875;0.21040098232099191388755343723460100591182708740234375;-0.737539537450413451580288892728276550769805908203125;0.60486038776342831990717741064145229756832122802734375]
      mask Display: e = 0.06;c1 = [120 150 230]/255;c2 = ([120 150 230]+0)/383;c3 = ([120 150 230]+128)/383;patch([0 1 1 0],[0 0 1 1],c1);patch([0 1 1 1-e 1-e 0+e],[0 0 1 1-e 0+e 0+e],c2);patch([0 0 1 1-e 0+e 0+e],[0 1 1 1-e 1-e 0+e],c3);plot([0 1 1 0 0],[0 0 1 1 0]);disp('weights');
  "IW{3,2}(3,:)'" : Constant  Value=[0.07347467212668712388534686397179029881954193115234375;0.7861108868576864860955311087309382855892181396484375;-0.67566774572860432979126699137850664556026458740234375;-0.458835457256843104456578430472291074693202972412109375;-0.55707982842666303735512656203354708850383758544921875;0.8719477238009958330877680054982192814350128173828125;0.495561359403498158382461724613676778972148895263671875;-0.3564291667486239045814500059350393712520599365234375;-0.641739480431748443578499063733033835887908935546875;0.195995587998245290872745272281463257968425750732421875;-0.5343802070489880318149289450957439839839935302734375;0.5914986515266236200005778300692327320575714111328125;0.76475314430197116610798957481165416538715362548828125;0.2299721294319108100268067573779262602329254150390625;-0.865019843509569508199774645618163049221038818359375]
      mask Display: e = 0.06;c1 = [120 150 230]/255;c2 = ([120 150 230]+0)/383;c3 = ([120 150 230]+128)/383;patch([0 1 1 0],[0 0 1 1],c1);patch([0 1 1 1-e 1-e 0+e],[0 0 1 1-e 0+e 0+e],c2);patch([0 0 1 1-e 0+e 0+e],[0 1 1 1-e 1-e 0+e],c3);plot([0 1 1 0 0],[0 0 1 1 0]);disp('weights');
  "IW{3,2}(4,:)'" : Constant  Value=[0.5432689582091401181429546340950764715671539306640625;-0.34639694789762831561574785155244171619415283203125;-0.263628299585251302250554772399482317268848419189453125;-1.0052764521815398257587048647110350430011749267578125;-0.41214491961734400771177888600504957139492034912109375;0.7124209955475444555617059450014494359493255615234375;0.409189441710246182282162408228032290935516357421875;-0.6636546541539967147826928339782170951366424560546875;0.053461019622592316491438424463922274298965930938720703125;0.5690138549430006076335075704264454543590545654296875;0.8077109987031387827727257899823598563671112060546875;1.0992513690498377787463368804310448467731475830078125;-0.34112217054730986642852030854555778205394744873046875;-0.37985793570625581150324023838038556277751922607421875;0.59612395242443405596333150242571718990802764892578125]
      mask Display: e = 0.06;c1 = [120 150 230]/255;c2 = ([120 150 230]+0)/383;c3 = ([120 150 230]+128)/383;patch([0 1 1 0],[0 0 1 1],c1);patch([0 1 1 1-e 1-e 0+e],[0 0 1 1-e 0+e 0+e],c2);patch([0 0 1 1-e 0+e 0+e],[0 1 1 1-e 1-e 0+e],c3);plot([0 1 1 0 0],[0 0 1 1 0]);disp('weights');
  "IW{3,2}(5,:)'" : Constant  Value=[-0.3588509129489612092811512411572039127349853515625;-0.2134984693101402708492742021917365491390228271484375;-0.5743803120801260764238804767956025898456573486328125;-0.3494457308399512296404054723097942769527435302734375;0.6888847366038770569929283738019876182079315185546875;0.6438233246750513227851797637413255870342254638671875;0.4343864929782539352487447104067541658878326416015625;0.8299335012373145747943681271863169968128204345703125;-0.977740199254297781550349100143648684024810791015625;-0.1743440358086640884494045167230069637298583984375;-0.4894708103269522769807053919066675007343292236328125;-0.476294769714211696509664761833846569061279296875;-0.1289174049630747997952084915596060454845428466796875;-0.6073704319228740988734216443845070898532867431640625;0.4184468226478561536652023278293199837207794189453125]
      mask Display: e = 0.06;c1 = [120 150 230]/255;c2 = ([120 150 230]+0)/383;c3 = ([120 150 230]+128)/383;patch([0 1 1 0],[0 0 1 1],c1);patch([0 1 1 1-e 1-e 0+e],[0 0 1 1-e 0+e 0+e],c2);patch([0 0 1 1-e 0+e 0+e],[0 1 1 1-e 1-e 0+e],c3);plot([0 1 1 0 0],[0 0 1 1 0]);disp('weights');
  "IW{3,2}(6,:)'" : Constant  Value=[-0.378010270755474220294445331091992557048797607421875;-0.11458975423711863228515284163222531788051128387451171875;0.011643142662950578536396051276824437081813812255859375;0.07901737914990382416480230176603072322905063629150390625;0.8868992949052956209499143369612284004688262939453125;-0.037586453998124103037525856052525341510772705078125;-0.1803775925809176505776321164375985972583293914794921875;-0.323661141390165274511758752851164899766445159912109375;-0.09220585109959249237032707924299756996333599090576171875;-0.616850147911289781177401891909539699554443359375;-0.94474850143867872276359776151366531848907470703125;0.2458835348049766000855242964462377130985260009765625;-0.78770050318993067861583767808042466640472412109375;-0.2324012163976034439638596040822449140250682830810546875;0.420797842904295615884535664008581079542636871337890625]
      mask Display: e = 0.06;c1 = [120 150 230]/255;c2 = ([120 150 230]+0)/383;c3 = ([120 150 230]+128)/383;patch([0 1 1 0],[0 0 1 1],c1);patch([0 1 1 1-e 1-e 0+e],[0 0 1 1-e 0+e 0+e],c2);patch([0 0 1 1-e 0+e 0+e],[0 1 1 1-e 1-e 0+e],c3);plot([0 1 1 0 0],[0 0 1 1 0]);disp('weights');
  "IW{3,2}(7,:)'" : Constant  Value=[-0.736225532853444608605286703095771372318267822265625;-0.8448614327930956680035023964592255651950836181640625;0.041670450798830256655680415178721887059509754180908203125;0.67546345257746642776197631974355317652225494384765625;0.46907615211557607270975722713046707212924957275390625;0.50057558032053339758249421720393002033233642578125;0.5798313036631512762397733240504749119281768798828125;-0.8785823689008938064404219403513707220554351806640625;0.5185294669844064952002327117952518165111541748046875;-0.377963130146548309529208609092165715992450714111328125;-0.215501408528878446446697125793434679508209228515625;-0.57465458199555019547233314369805157184600830078125;0.1420123850784229257993018791239592246711254119873046875;-0.5856362431238864019178436137735843658447265625;0.294704176863094302607493091272772289812564849853515625]
      mask Display: e = 0.06;c1 = [120 150 230]/255;c2 = ([120 150 230]+0)/383;c3 = ([120 150 230]+128)/383;patch([0 1 1 0],[0 0 1 1],c1);patch([0 1 1 1-e 1-e 0+e],[0 0 1 1-e 0+e 0+e],c2);patch([0 0 1 1-e 0+e 0+e],[0 1 1 1-e 1-e 0+e],c3);plot([0 1 1 0 0],[0 0 1 1 0]);disp('weights');
  "IW{3,2}(8,:)'" : Constant  Value=[0.6659111033267490764586682416847907006740570068359375;0.7810742177994451918010554436477832496166229248046875;-0.8862999566675682228122923334012739360332489013671875;0.54758572404517569243154184732702560722827911376953125;0.1616798707065492113343907476519234478473663330078125;0.6800985344857626291315000344184227287769317626953125;-0.409683730537387436054785894157248549163341522216796875;-0.23535436306165091746578355014207772910594940185546875;-0.818615371547309234045997072826139628887176513671875;0.568105080532512740632000713958404958248138427734375;0.644081626596956891006584555725567042827606201171875;-0.81562062570170701381044864319846965372562408447265625;-0.26341296674659198107093516227905638515949249267578125;-0.88001813315795296421839566392009146511554718017578125;0.06255802736854450263326299364052829332649707794189453125]
      mask Display: e = 0.06;c1 = [120 150 230]/255;c2 = ([120 150 230]+0)/383;c3 = ([120 150 230]+128)/383;patch([0 1 1 0],[0 0 1 1],c1);patch([0 1 1 1-e 1-e 0+e],[0 0 1 1-e 0+e 0+e],c2);patch([0 0 1 1-e 0+e 0+e],[0 1 1 1-e 1-e 0+e],c3);plot([0 1 1 0 0],[0 0 1 1 0]);disp('weights');
  "IW{3,2}(9,:)'" : Constant  Value=[-0.406402272703359546124346479700761847198009490966796875;0.78023986432559866432967510263551957905292510986328125;-0.91749834749657221966145925762248225510120391845703125;0.266390133198962486549277173253358341753482818603515625;-0.0060882964218065271921886960626579821109771728515625;0.259130345430842456977416077279485762119293212890625;0.159611063762088944972816761946887709200382232666015625;-0.71883191289486358943605637250584550201892852783203125;0.323093600384308177186909460942842997610569000244140625;-0.54283720388258827060923294993699528276920318603515625;0.095411385035422568989815772511065006256103515625;0.44335877624726283130485171568579971790313720703125;-0.11990503822457691807112922788292053155601024627685546875;0.69037926136484173422758203741977922618389129638671875;0.69920759623566441920416991706588305532932281494140625]
      mask Display: e = 0.06;c1 = [120 150 230]/255;c2 = ([120 150 230]+0)/383;c3 = ([120 150 230]+128)/383;patch([0 1 1 0],[0 0 1 1],c1);patch([0 1 1 1-e 1-e 0+e],[0 0 1 1-e 0+e 0+e],c2);patch([0 0 1 1-e 0+e 0+e],[0 1 1 1-e 1-e 0+e],c3);plot([0 1 1 0 0],[0 0 1 1 0]);disp('weights');
  Mux : Mux  Inputs=15
      mask Display: e = 0.06;c1 = [120 150 230]/255;c2 = ([120 150 230]+0)/383;c3 = ([120 150 230]+128)/383;patch([0 1 1 0],[0 0 1 1],c1);patch([0 1 1 1-e 1-e 0+e],[0 0 1 1-e 0+e 0+e],c2);patch([0 0 1 1-e 0+e 0+e],[0 1 1 1-e 1-e 0+e],c3);plot([0 1 1 0 0],[0 0 1 1 0]);disp('Mux');
  dotprod{1..15} (15 alike) : neural/Weight Functions/dotprod
  "lz{3,2}" : Outport
      mask Display: e = 0.06;c1 = [120 230 180]/255;c2 = ([120 230 180]+0)/(256+128);c3 = ([120 230 180]+128)/(256+128);patch([0 1 1 0],[0 0 1 1],c1);patch([0 1 1 1-e 1-e 0+e],[0 0 1 1-e 0+e 0+e],c2);patch([0 0 1 1-e 0+e 0+e],[0 1 1 1-e 1-e 0+e],c3);plot([0 1 1 0 0],[0 0 1 1 0]);
  wires:
  "IW{3,2}(1,:)'"/1 -> dotprod1/1
  "ad{3,2}"/1 -> dotprod1/2, dotprod2/2, dotprod3/2, dotprod4/2, dotprod5/2, dotprod6/2, dotprod7/2, dotprod8/2, dotprod9/2, dotprod10/2, dotprod11/2, dotprod12/2, dotprod13/2, dotprod14/2, dotprod15/2
  dotprod1/1 -> Mux/1
  "IW{3,2}(2,:)'"/1 -> dotprod2/1
  dotprod2/1 -> Mux/2
  "IW{3,2}(3,:)'"/1 -> dotprod3/1
  dotprod3/1 -> Mux/3
  "IW{3,2}(4,:)'"/1 -> dotprod4/1
  dotprod4/1 -> Mux/4
  "IW{3,2}(5,:)'"/1 -> dotprod5/1
  dotprod5/1 -> Mux/5
  "IW{3,2}(6,:)'"/1 -> dotprod6/1
  dotprod6/1 -> Mux/6
  "IW{3,2}(7,:)'"/1 -> dotprod7/1
  dotprod7/1 -> Mux/7
  "IW{3,2}(8,:)'"/1 -> dotprod8/1
  dotprod8/1 -> Mux/8
  "IW{3,2}(9,:)'"/1 -> dotprod9/1
  dotprod9/1 -> Mux/9
  "IW{3,2}(10,:)'"/1 -> dotprod10/1
  dotprod10/1 -> Mux/10
  "IW{3,2}(11,:)'"/1 -> dotprod11/1
  dotprod11/1 -> Mux/11
  "IW{3,2}(12,:)'"/1 -> dotprod12/1
  dotprod12/1 -> Mux/12
  "IW{3,2}(13,:)'"/1 -> dotprod13/1
  dotprod13/1 -> Mux/13
  "IW{3,2}(14,:)'"/1 -> dotprod14/1
  dotprod14/1 -> Mux/14
  "IW{3,2}(15,:)'"/1 -> dotprod15/1
  dotprod15/1 -> Mux/15
  Mux/1 -> "lz{3,2}"/1

== system AFC_FFNN_trainlm_15_15_15_15_Apr_1_2020/Air Fuel Control Model 1/Feed-Forward Neural Network/Layer 4/Delays 1 ==
  "p{4}" : Inport  PortDimensions=15
      mask Display: e = 0.06;c1 = [120 230 180]/255;c2 = ([120 230 180]+0)/(256+128);c3 = ([120 230 180]+128)/(256+128);patch([0 1 1 0],[0 0 1 1],c1);patch([0 1 1 1-e 1-e 0+e],[0 0 1 1-e 0+e 0+e],c2);patch([0 0 1 1-e 0+e 0+e],[0 1 1 1-e 1-e 0+e],c3);plot([0 1 1 0 0],[0 0 1 1 0]);
  mux : Mux  Inputs=1
      mask Display: e = 0.06;c1 = [120 150 230]/255;c2 = ([120 150 230]+0)/383;c3 = ([120 150 230]+128)/383;patch([0 1 1 0],[0 0 1 1],c1);patch([0 1 1 1-e 1-e 0+e],[0 0 1 1-e 0+e 0+e],c2);patch([0 0 1 1-e 0+e 0+e],[0 1 1 1-e 1-e 0+e],c3);plot([0 1 1 0 0],[0 0 1 1 0]);disp('Mux')
  "pd{4,3}" : Outport
      mask Display: e = 0.06;c1 = [120 230 180]/255;c2 = ([120 230 180]+0)/(256+128);c3 = ([120 230 180]+128)/(256+128);patch([0 1 1 0],[0 0 1 1],c1);patch([0 1 1 1-e 1-e 0+e],[0 0 1 1-e 0+e 0+e],c2);patch([0 0 1 1-e 0+e 0+e],[0 1 1 1-e 1-e 0+e],c3);plot([0 1 1 0 0],[0 0 1 1 0]);
  wires:
  "p{4}"/1 -> mux/1
  mux/1 -> "pd{4,3}"/1
